simulink model "quad_system_3"  (R2023a)
settings: Solver=VariableStepAuto  StartTime=0.0  StopTime=40  RelTol=1e-7
InitFcn:
  | % quadrotor parameters
  | m = 1;
  | C = 1;
  | J_phi = 1;
  | l = 1;
  | J_theta = 1;
  | J_psi = 1;
  | M = blkdiag(1/m,C/J_phi,l/J_theta,l/J_psi);
  | g = 9.81;
  | 
  | % controller parameters
  | kappa = 100;
  | a_1 = 5;
  | a_2 = 10;
  | a_3 = 10;
  | a_4 = 5;
  | a_5 = 1;
  | %kappa = 100;
  | %a_1 = 5;
  | %a_2 = 10;
  | %a_3 = 10;
  | %a_4 = 5;
  | %a_5 = 1;
  | gamma_1 = 1;
  | gamma_2 = 4;
  | gamma_3 = 6;
  | gamma_4 = 4;
  | L = 5;
  | ell = 0.9;
settings Model: Creator=Dell  LastModifiedBy=Dell
settings DebuggingCC: UnconnectedInputMsg=warning  UnconnectedOutputMsg=warning  UnconnectedLineMsg=warning
settings ModelReferenceCC: EnableRefExpFcnMdlSchedulingChecks=on
settings RTWCC: DLArmComputeVersion=19.05

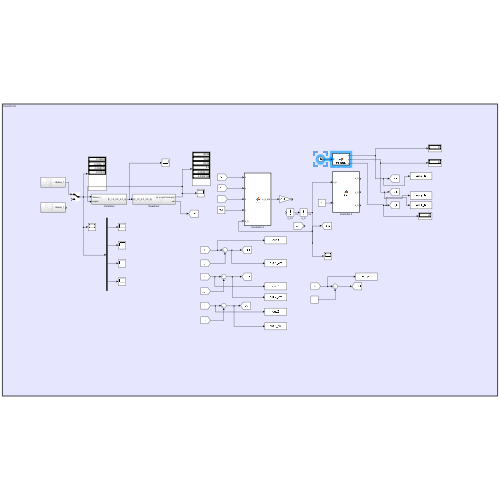
[thumbnail: Simulink's stored preview of the top-level diagram]
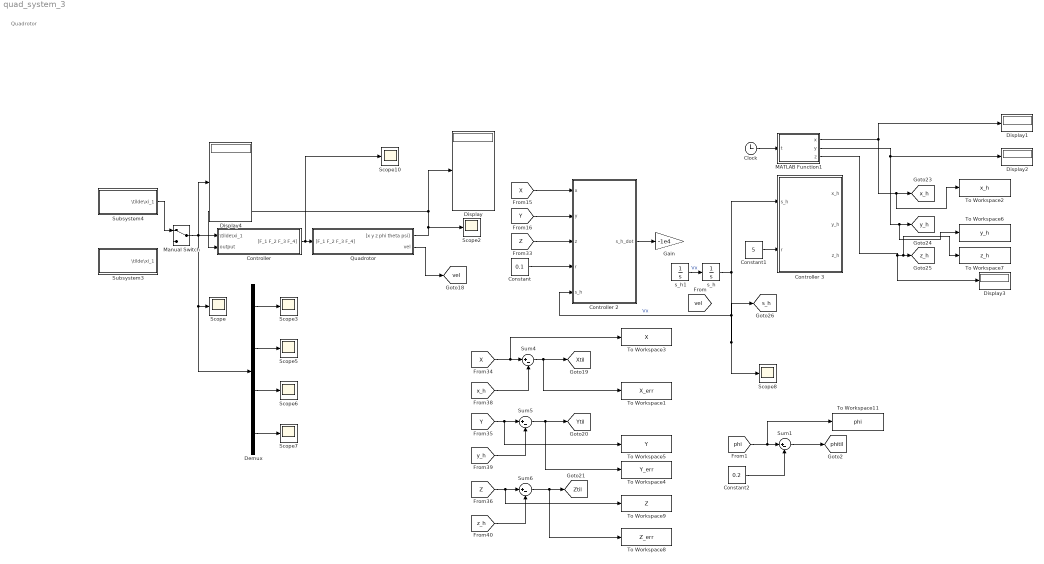
== system quad_system_3 ==
  note: Quadrotor
  Clock : Clock
  Constant : Constant  Value=0.1
  Constant1 : Constant  Value=5
  Constant2 : Constant  Value=0.2
  Controller : Subsystem
  Controller 2 : MATLAB Function  TreatAsAtomicUnit=on
  Controller 3 : MATLAB Function  TreatAsAtomicUnit=on
  Demux : Demux
  Display{,1..4} (5 alike) : Display
  Gain : Gain  Gain=-1e4
  MATLAB Function1 : MATLAB Function  TreatAsAtomicUnit=on
  Manual Switch : ManualSwitch
  Quadrotor : Subsystem
  Scope{,2..3,5..8,10} (8 alike) : Scope
  Subsystem3 : Subsystem
  Subsystem4 : Subsystem
  Sum{1,4..6} (4 alike) : Sum  Inputs=|+-
  To Workspace1 : ToWorkspace  VariableName=X_err  SaveFormat=Timeseries  SampleTime=-1
  To Workspace11 : ToWorkspace  VariableName=phi  SaveFormat=Structure With Time  SampleTime=-1
  To Workspace2 : ToWorkspace  VariableName=x_h  SaveFormat=Timeseries  SampleTime=-1
  To Workspace3 : ToWorkspace  VariableName=X  SaveFormat=Timeseries  SampleTime=-1
  To Workspace4 : ToWorkspace  VariableName=Y_err  SaveFormat=Timeseries  SampleTime=-1
  To Workspace5 : ToWorkspace  VariableName=Y  SaveFormat=Timeseries  SampleTime=-1
  To Workspace6 : ToWorkspace  VariableName=y_h  SaveFormat=Timeseries  SampleTime=-1
  To Workspace7 : ToWorkspace  VariableName=z_h  SaveFormat=Timeseries  SampleTime=-1
  To Workspace8 : ToWorkspace  VariableName=Z_err  SaveFormat=Timeseries  SampleTime=-1
  To Workspace9 : ToWorkspace  VariableName=Z  SaveFormat=Timeseries  SampleTime=-1
  s_h : Integrator  InitialCondition=2/3
  s_h1 : Integrator  InitialCondition=1
  tag scope: Xtil=global, Ytil=global, Ztil=global, phitil=global, s_h=global, vel=global, x_h=global, y_h=global, z_h=global
  wires:
  [y_h] -> Sum5/2
  Quadrotor/2(vel) -> [vel]
  s_h/1 -> Scope8/1, [s_h], Controller 2/5(s_h), Controller 3/1(s_h)  "Vx"
  [z_h] -> Sum6/2
  MATLAB Function1/2(y) -> To Workspace6/1, [y_h], Display2/1
  Quadrotor/1("[x y z phi theta psi]") -> Display/1, Controller/2(output), Scope2/1
  Sum4/1 -> To Workspace1/1, [Xtil]
  Controller/1("[F_1 F_2 F_3 F_4]") -> Scope10/1, Quadrotor/1("[F_1 F_2 F_3 F_4]")
  Sum6/1 -> To Workspace8/1, [Ztil]
  [x_h] -> Sum4/2
  [X] -> To Workspace3/1, Sum4/1
  Controller 2/1(s_h_dot) -> Gain/1
  [Y] -> Controller 2/2(y)
  [Z] -> To Workspace9/1, Sum6/1
  Constant/1 -> Controller 2/4(r)
  Sum5/1 -> To Workspace4/1, [Ytil]
  Demux/2 -> Scope5/1
  [Y] -> To Workspace5/1, Sum5/1
  [Z] -> Controller 2/3(z)
  MATLAB Function1/3(z) -> Display3/1, To Workspace7/1, [z_h]
  Demux/4 -> Scope7/1
  Subsystem4/1(\tilde\xi_1) -> Manual Switch/1
  Demux/1 -> Scope3/1
  Constant1/1 -> Controller 3/2(r)
  Demux/3 -> Scope6/1
  MATLAB Function1/1(x) -> To Workspace2/1, [x_h], Display1/1
  s_h1/1 -> s_h/1  "Vx"
  Manual Switch/1 -> Display4/1, Controller/1(\tilde\xi_1), Demux/1, Scope/1
  [X] -> Controller 2/1(x)
  Constant2/1 -> Sum1/2
  [phi] -> To Workspace11/1, Sum1/1
  Sum1/1 -> [phitil]
  Clock/1 -> MATLAB Function1/1(t)

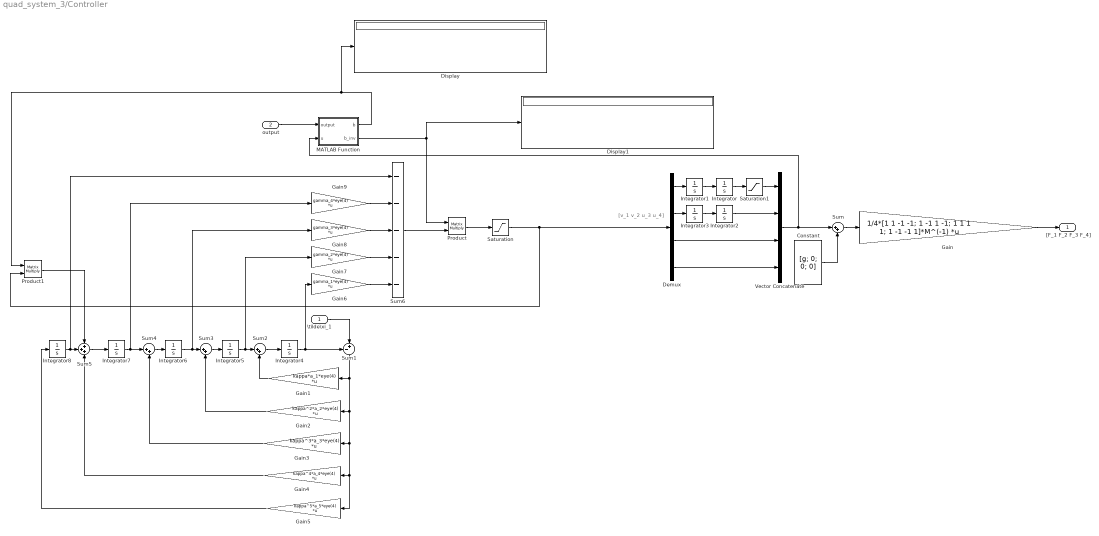
== system quad_system_3/Controller ==
  note: [v_1 v_2 u_3 u_4]
  \tilde\xi_1 : Inport
  output : Inport  Port=2
  Constant : Constant  Value=[g; 0; 0; 0]  VectorParams1D=off
  Demux : Demux
  Display : Display
  Display1 : Display
  Gain : Gain  Gain=1/4*[1 1 -1 -1; 1 -1 1 -1; 1 1 1 1; 1 -1 -1 1]*M^(-1)  Multiplication=Matrix(K*u) (u vector)
  Gain1 : Gain  Gain=kappa*a_1*eye(4)  Multiplication=Matrix(K*u) (u vector)
  Gain2 : Gain  Gain=kappa^2*a_2*eye(4)  Multiplication=Matrix(K*u) (u vector)
  Gain3 : Gain  Gain=kappa^3*a_3*eye(4)  Multiplication=Matrix(K*u) (u vector)
  Gain4 : Gain  Gain=kappa^4*a_4*eye(4)  Multiplication=Matrix(K*u) (u vector)
  Gain5 : Gain  Gain=kappa^5*a_5*eye(4)  Multiplication=Matrix(K*u) (u vector)
  Gain6 : Gain  Gain=gamma_1*eye(4)  Multiplication=Matrix(K*u) (u vector)
  Gain7 : Gain  Gain=gamma_2*eye(4)  Multiplication=Matrix(K*u) (u vector)
  Gain8 : Gain  Gain=gamma_3*eye(4)  Multiplication=Matrix(K*u) (u vector)
  Gain9 : Gain  Gain=gamma_4*eye(4)  Multiplication=Matrix(K*u) (u vector)
  Integrator{,1..8} (9 alike) : Integrator
  MATLAB Function : MATLAB Function  TreatAsAtomicUnit=on
  Product : Product  Multiplication=Matrix(*)
  Product1 : Product  Multiplication=Matrix(*)
  Saturation : Saturate  UpperLimit=L  LowerLimit=-L
  Saturation1 : Saturate  UpperLimit=ell*g  LowerLimit=-ell*g
  Sum{,2..4} (4 alike) : Sum  Inputs=|++
  Sum1 : Sum  Inputs=-+|
  Sum5 : Sum  Inputs=+++
  Sum6 : Sum  Inputs=-----
  Vector Concatenate : Concatenate  NumInputs=4
  "[F_1 F_2 F_3 F_4]" : Outport
  wires:
  Gain/1 -> "[F_1 F_2 F_3 F_4]"/1
  Sum/1 -> Gain/1
  Constant/1 -> Sum/2
  Integrator1/1 -> Integrator/1
  Integrator3/1 -> Integrator2/1
  Integrator/1 -> Saturation1/1
  Integrator2/1 -> Vector Concatenate/2
  Demux/1 -> Integrator1/1
  Demux/2 -> Integrator3/1
  Demux/3 -> Vector Concatenate/3
  Demux/4 -> Vector Concatenate/4
  Vector Concatenate/1 -> MATLAB Function/2(u), Sum/1
  Integrator4/1 -> Sum1/1, Gain6/1
  \tilde\xi_1/1 -> Sum1/2
  Sum1/1 -> Gain5/1, Gain4/1, Gain3/1, Gain2/1, Gain1/1
  Gain1/1 -> Sum2/2
  Sum2/1 -> Integrator4/1
  Integrator5/1 -> Gain7/1, Sum2/1
  Sum3/1 -> Integrator5/1
  Gain2/1 -> Sum3/2
  Integrator6/1 -> Gain8/1, Sum3/1
  Sum4/1 -> Integrator6/1
  Gain3/1 -> Sum4/2
  Integrator7/1 -> Gain9/1, Sum4/1
  Sum5/1 -> Integrator7/1
  Gain4/1 -> Sum5/3
  Integrator8/1 -> Sum6/1, Sum5/2
  Gain5/1 -> Integrator8/1
  Gain6/1 -> Sum6/5
  Gain7/1 -> Sum6/4
  Gain8/1 -> Sum6/3
  Gain9/1 -> Sum6/2
  Sum6/1 -> Product/2
  Product/1 -> Saturation/1
  Product1/1 -> Sum5/1
  MATLAB Function/2(b_inv) -> Display1/1, Product/1
  MATLAB Function/1(b) -> Product1/1, Display/1
  output/1 -> MATLAB Function/1(output)
  Saturation/1 -> Product1/2, Demux/1
  Saturation1/1 -> Vector Concatenate/1

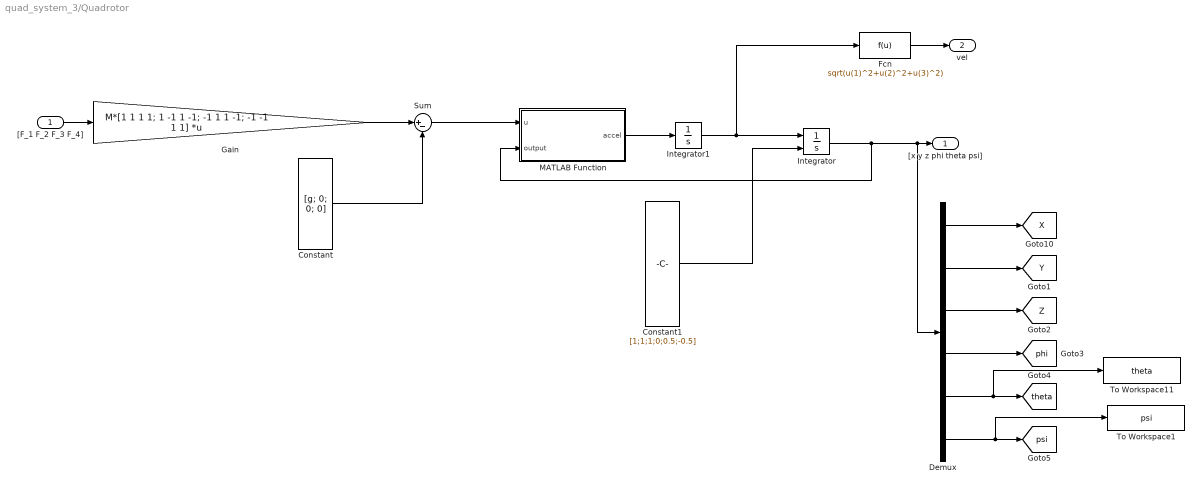
== system quad_system_3/Quadrotor ==
  "[F_1 F_2 F_3 F_4]" : Inport
  Constant : Constant  Value=[g; 0; 0; 0]  VectorParams1D=off
  Constant1 : Constant  Value=[1;1;1;0;0.5;-0.5]  VectorParams1D=off
  Demux : Demux  Outputs=6
  Fcn : Fcn  Expr=sqrt(u(1)^2+u(2)^2+u(3)^2)
  Gain : Gain  Gain="M*[1 1 1 1; 1 -1 1 -1; -1 1 1 -1;  -1 -1 1 1]"  Multiplication=Matrix(K*u) (u vector)
  Integrator : Integrator  InitialConditionSource=external  InitialCondition=[0;1;1;1;0;0]
  Integrator1 : Integrator
  MATLAB Function : MATLAB Function  TreatAsAtomicUnit=on
  Sum : Sum  Inputs=|+-
  To Workspace1 : ToWorkspace  VariableName=psi  SaveFormat=Structure With Time  SampleTime=-1
  To Workspace11 : ToWorkspace  VariableName=theta  SaveFormat=Structure With Time  SampleTime=-1
  "[x y z phi theta psi]" : Outport
  vel : Outport  Port=2
  tag scope: X=global, Y=global, Z=global, phi=global, psi=global, theta=global
  wires:
  Integrator1/1 -> Fcn/1, Integrator/1
  Integrator/1 -> Demux/1, "[x y z phi theta psi]"/1, MATLAB Function/2(output)
  MATLAB Function/1(accel) -> Integrator1/1
  "[F_1 F_2 F_3 F_4]"/1 -> Gain/1
  Gain/1 -> Sum/1
  Constant/1 -> Sum/2
  Sum/1 -> MATLAB Function/1(u)
  Constant1/1 -> Integrator/2
  Demux/1 -> [X]
  Demux/2 -> [Y]
  Demux/3 -> [Z]
  Demux/4 -> [phi]
  Demux/5 -> To Workspace11/1, [theta]
  Demux/6 -> To Workspace1/1, [psi]
  Fcn/1 -> vel/1

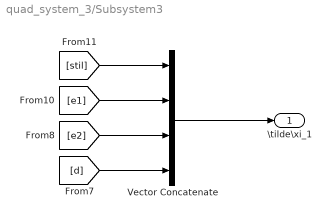
== system quad_system_3/Subsystem3 ==
  Vector Concatenate : Concatenate  NumInputs=4
  \tilde\xi_1 : Outport
  wires:
  [e1] -> Vector Concatenate/2
  [stil] -> Vector Concatenate/1
  [e2] -> Vector Concatenate/3
  Vector Concatenate/1 -> \tilde\xi_1/1
  [d] -> Vector Concatenate/4

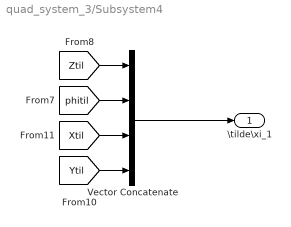
== system quad_system_3/Subsystem4 ==
  Vector Concatenate : Concatenate  NumInputs=4
  \tilde\xi_1 : Outport
  wires:
  Vector Concatenate/1 -> \tilde\xi_1/1
  [Ztil] -> Vector Concatenate/1
  [phitil] -> Vector Concatenate/2
  [Xtil] -> Vector Concatenate/3
  [Ytil] -> Vector Concatenate/4

== matlab function quad_system_3/Controller/MATLAB Function ==
  data: output input; u input; b output; b_inv output
function [b,b_inv] = fcn(output,u)

no = 0;
simple = 1;
full = 2;

flag = full;

phi = output(4);

theta = output(5);

psi = output(6);

ct = cos(theta);
st = sin(theta);

cp = cos(psi);
sp = sin(psi);

g = 9.81;
d = u(1)+g;

if flag == simple
b = [1 0 0 0; 
     0 1 0 0; 
     0 0 cos(phi)*d sin(phi)*d; 
     0 0 sin(phi)*d -cos(phi)*d];
elseif flag == full
b = [1 0 0 0; 
     0 1 0 0; 
     0 0 cos(phi) -sin(phi); 
     0 0 sin(phi) cos(phi)]*...
    [ct*cp 0 -st*cp*d -ct*sp*d ; 
     0 1 0 0;
     st*cp 0 ct*cp*d -st*sp*d;
     -sp 0 0 -cp*d];
else 
    b =eye(4);
end

b_inv  = inv(b);

== matlab function quad_system_3/MATLAB Function1 ==
  data: x output; t input; y output; z output
function [x, y, z] = trajectory(t)
    % Определение ориентиров A, B, C, D
    A = [5, 5, 5];
    B = [10, 10, 5];
    C = [20, 5, 10];
    D = [30, 20, 20];

    % Объединяем ориентиры в матрицу
    waypoints = [A; B; C; D]; 
    % Время достижения ориентиров
    t_waypoints = [5; 10; 20; 30];

    % Интерполяция
    if t < t_waypoints(1)
        % Если время меньше первого ориентира
        x = A(1);
        y = A(2);
        z = A(3);
    elseif t > t_waypoints(end)
        % Если время больше последнего ориентира
        x = D(1);
        y = D(2);
        z = D(3);
    else
        % Линейная интерполяция по x, y и z
        x = interp1(t_waypoints, waypoints(:,1), t, 'linear'); 
        y = interp1(t_waypoints, waypoints(:,2), t, 'linear'); 
        z = interp1(t_waypoints, waypoints(:,3), t, 'linear'); 
    end
end

== matlab function quad_system_3/Controller 2 ==
  data: x input; y input; z input; r input; s_h_dot output; s_h input
function s_h_dot   = fcn(x,y,z,r,s_h)


rho = 1;
H = 5*s_h - x - y - z;

%rho = 1 + r*cos(s_h)*x + r*sin(s_h)*y;

%H = r*sin(s_h)*x - r*cos(s_h)*y - z + s_h;

s_h_dot = rho*H;

== matlab function quad_system_3/Controller 3 ==
  data: s_h input; r input; x_h output; y_h output; z_h output
function [x_h,y_h,z_h]= fcn(s_h, r)
x_h = r * cos(s_h);

y_h = r* sin(s_h);

z_h = s_h;
end

== matlab function quad_system_3/Quadrotor/MATLAB Function ==
  data: u input; accel output; output input
function accel = fcn(u, output)

g = 9.81;
phi = output(4);
theta = output(5);
psi = output(6);

accel_lin = [cos(phi)*sin(theta)*cos(psi)+sin(phi)*sin(psi);...
    sin(phi)*sin(theta)*cos(psi)-cos(phi)*sin(psi);...
    cos(theta)*cos(psi)]*(u(1)+g)-[0; 0; g];

accel_ang = [u(2); u(3); u(4)];

accel = [accel_lin; accel_ang];
